simulink model "tpscode"  (R2022b)
settings: Solver=FixedStepDiscrete  StartTime=0.0  StopTime=10.0  FixedStep=1e-3  RelTol=1e-3
undefined symbols (not defined in the file): TPS_Modes
settings Model: Creator=ahmed  LastModifiedBy=ahmed
settings OptimizationCC: DefaultParameterBehavior=Inlined  UseDivisionForNetSlopeComputation=on  GainParamInheritBuiltInType=on  UseFloatMulNetSlope=on  InlineInvariantSignals=on  PassReuseOutputArgsAs=Individual arguments  ZeroExternalMemoryAtStartup=off  ZeroInternalMemoryAtStartup=off  NoFixptDivByZeroProtection=on  EfficientFloat2IntCast=on  LifeSpan=1  OptimizeBlockOrder=speed  DifferentSizesBufferReuse=on  EfficientTunableParamExpr=on
settings DebuggingCC: ParameterTunabilityLossMsg=error
settings HardwareCC: ProdBitPerInt=16  ProdBitPerPointer=16  ProdBitPerSizeT=16  ProdBitPerPtrDiffT=16  ProdLargestAtomicFloat=None  ProdWordSize=16  ProdLongLongMode=on  ProdHWDeviceType=Atmel->AVR (8-bit)
settings SFSimCC: MATLABDynamicMemAlloc=off
settings RTWCC: Description=Embedded Coder  SystemTargetFile=ert.tlc  TemplateMakefile=ert_default_tmf
settings CodeAppCC: ForceParamTrailComments=on  IgnoreCustomStorageClasses=off  OperatorAnnotations=on  SimulinkDataObjDesc=on  SFDataObjDesc=on  CustomSymbolStrGlobalVar=rt$N$M  CustomSymbolStrType=$N$M  CustomSymbolStrFcn=$N$M$F  CustomSymbolStrMacro=$N$M  InsertBlockDesc=on
settings ERTTargetCC: TargetLangStandard=C99 (ISO)  GenerateSampleERTMain=on  IncludeMdlTerminateFcn=off  CombineSignalStateStructs=on  SuppressErrorStatus=on  SupportAbsoluteTime=off  PurelyIntegerCode=on  SupportNonFinite=off  SupportComplex=off  InlinedParameterPlacement=NonHierarchical  ERTCustomFileTemplate=example_file_process.tlc  ERTFilePackagingFormat=CompactWithDataFile

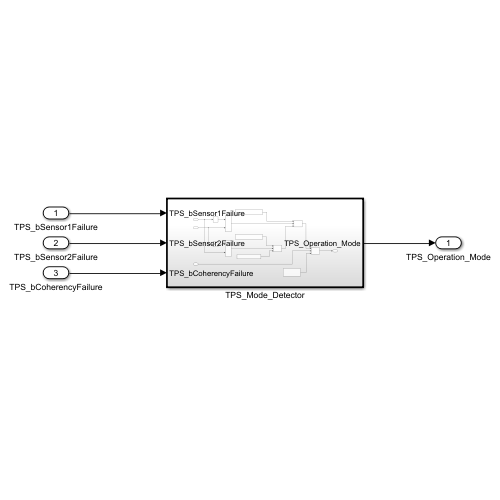
[thumbnail: Simulink's stored preview of the top-level diagram]
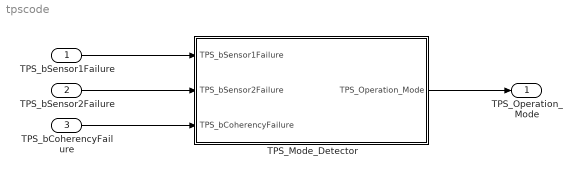
== system tpscode ==
  TPS_bSensor1Failure : Inport  OutDataTypeStr=boolean
  TPS_bSensor2Failure : Inport  Port=2  OutDataTypeStr=boolean
  TPS_bCoherencyFailure : Inport  Port=3  OutDataTypeStr=boolean
  TPS_Mode_Detector : Subsystem  TreatAsAtomicUnit=on
  TPS_Operation_Mode : Outport  OutDataTypeStr=Enum: TPS_Modes
  wires:
  TPS_bSensor1Failure/1 -> TPS_Mode_Detector/1(TPS_bSensor1Failure)
  TPS_bSensor2Failure/1 -> TPS_Mode_Detector/2(TPS_bSensor2Failure)
  TPS_Mode_Detector/1(TPS_Operation_Mode) -> TPS_Operation_Mode/1
  TPS_bCoherencyFailure/1 -> TPS_Mode_Detector/3(TPS_bCoherencyFailure)

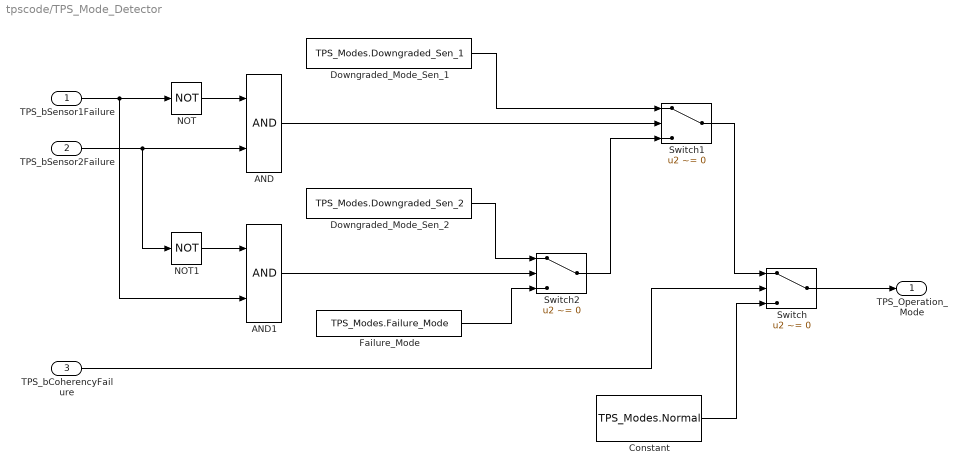
== system tpscode/TPS_Mode_Detector ==
  TPS_bSensor1Failure : Inport  OutDataTypeStr=boolean
  TPS_bSensor2Failure : Inport  Port=2  OutDataTypeStr=boolean
  TPS_bCoherencyFailure : Inport  Port=3  OutDataTypeStr=boolean
  AND : Logic  AllPortsSameDT=off  OutDataTypeStr=boolean
  AND1 : Logic  AllPortsSameDT=off  OutDataTypeStr=boolean
  Constant : Constant  Value=TPS_Modes.Normal
  Downgraded_Mode_Sen_1 : Constant  Value=TPS_Modes.Downgraded_Sen_1
  Downgraded_Mode_Sen_2 : Constant  Value=TPS_Modes.Downgraded_Sen_2
  Failure_Mode : Constant  Value=TPS_Modes.Failure_Mode
  NOT : Logic  Operator=NOT  AllPortsSameDT=off  OutDataTypeStr=boolean
  NOT1 : Logic  Operator=NOT  AllPortsSameDT=off  OutDataTypeStr=boolean
  Switch : Switch  Criteria=u2 ~= 0  SaturateOnIntegerOverflow=off  InputSameDT=off
  Switch1 : Switch  Criteria=u2 ~= 0  SaturateOnIntegerOverflow=off  InputSameDT=off
  Switch2 : Switch  Criteria=u2 ~= 0  SaturateOnIntegerOverflow=off  InputSameDT=off
  TPS_Operation_Mode : Outport  OutDataTypeStr=Enum: TPS_Modes
  wires:
  TPS_bCoherencyFailure/1 -> Switch/2
  Constant/1 -> Switch/3
  TPS_bSensor1Failure/1 -> NOT/1, AND1/2
  NOT/1 -> AND/1
  TPS_bSensor2Failure/1 -> AND/2, NOT1/1
  AND/1 -> Switch1/2
  Downgraded_Mode_Sen_1/1 -> Switch1/1
  NOT1/1 -> AND1/1
  Downgraded_Mode_Sen_2/1 -> Switch2/1
  AND1/1 -> Switch2/2
  Failure_Mode/1 -> Switch2/3
  Switch2/1 -> Switch1/3
  Switch1/1 -> Switch/1
  Switch/1 -> TPS_Operation_Mode/1
